simulink model "simulacao_mod_discr"  (R2012b)
settings: Solver=ode3  StartTime=0.0  StopTime=3  FixedStep=1e-5  RelTol=1e-3
libraries: simulink x1
settings Model: Creator=h3now  LastModifiedBy=h3now

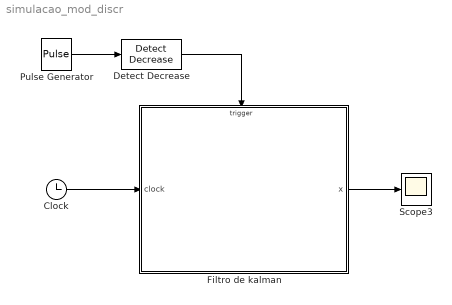
== system simulacao_mod_discr ==
  Clock : Clock
  Detect Decrease : simulink/Logic and Bit Operations/Detect Decrease  vinit=0.0  InputProcessing=Inherited  OutDataTypeStr=boolean
  Filtro de kalman : Subsystem
  Pulse Generator : DiscretePulseGenerator  PulseType=Time based  Period=0.004  PulseWidth=50
  Scope3 : Scope
      settings: ShowLegends=on  YMin=-50  YMax=50
  wires:
  Clock/1 -> Filtro de kalman/1(clock)
  Pulse Generator/1 -> Detect Decrease/1
  Detect Decrease/1 -> Filtro de kalman/Trigger
  Filtro de kalman/1(x) -> Scope3/1

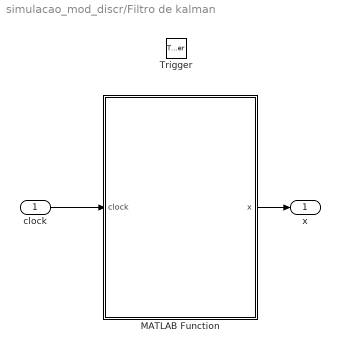
== system simulacao_mod_discr/Filtro de kalman ==
  clock : Inport
  Trigger : TriggerPort  PortDimensions=1
  MATLAB Function : MATLAB Function  TreatAsAtomicUnit=on
  x : Outport
  wires:
  clock/1 -> MATLAB Function/1(clock)
  MATLAB Function/1(x) -> x/1

== matlab function simulacao_mod_discr/Filtro de kalman/MATLAB Function ==
  data: x output; clock input
function x  = fcn(clock)
%#codegen

persistent t_old;
persistent x_posteriori_old;

if( isempty(t_old) || isempty(x_posteriori_old) )
    t_old = 0;
    x_posteriori_old = [200 0]';
end


deltaT = clock - t_old;
F = [1-435.7*deltaT -5067*deltaT ; deltaT 1];


% Previsão
x_priori = F * x_posteriori_old;


x_posteriori_old = x_priori;
t_old = clock;

x = x_priori;
